simulink model "fullproject"  (R2021b)
settings: Solver=VariableStepAuto  StartTime=0.0  StopTime=0.1  RelTol=1e-3
libraries: spsMeanLib x9, spsDiodeLib x7, spsSeriesRLCBranchLib x4, spsACVoltageSourceLib x3, spsCurrentMeasurementLib x3, spsVoltageMeasurementLib x3, spsDCVoltageSourceLib x2, spsIGBTLib x1, spspowerguiLib x1
settings Model: Creator=yorga  LastModifiedBy=mluser

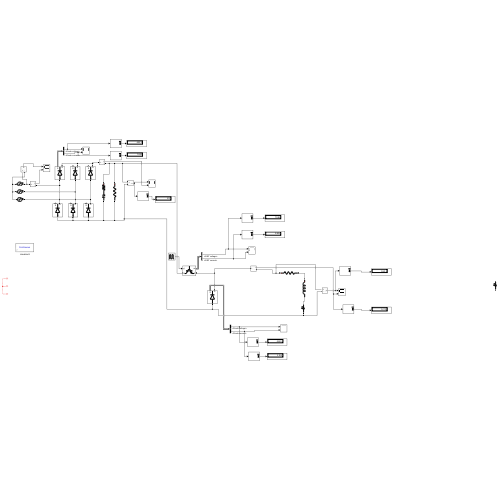
[thumbnail: Simulink's stored preview of the top-level diagram]
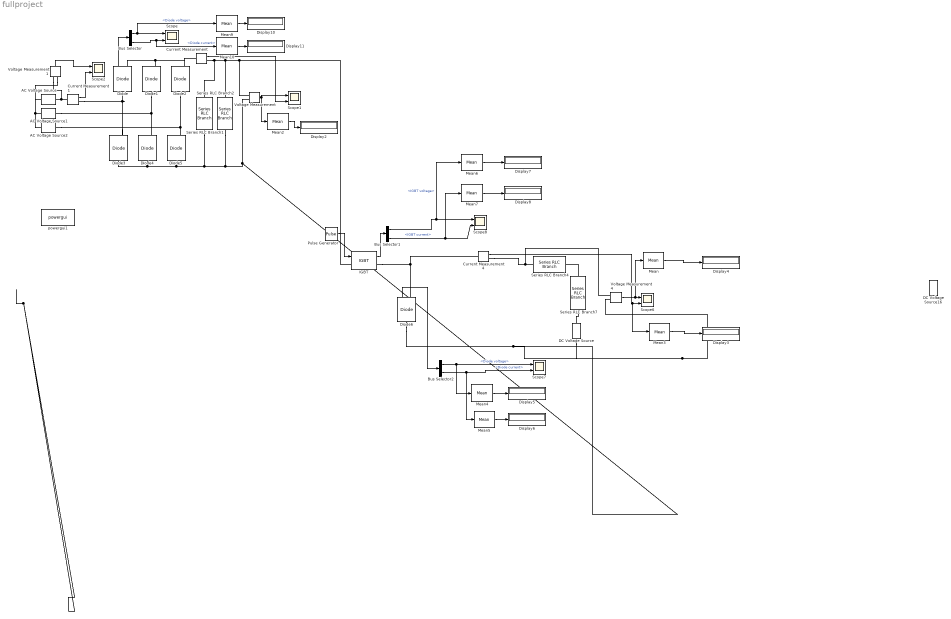
== system fullproject ==
  AC Voltage Source : spsACVoltageSourceLib/AC Voltage Source  Amplitude=100*sqrt(2)  Phase=0  Frequency=50  SampleTime=1e-4  Measurements=None  BusType=swing  Pref=10e3  Qref=0  Qmin=-inf  Qmax=+inf
  AC Voltage Source1 : spsACVoltageSourceLib/AC Voltage Source  Amplitude=100*sqrt(2)  Phase=-120  Frequency=50  SampleTime=1e-4  Measurements=None  BusType=swing  Pref=10e3  Qref=0  Qmin=-inf  Qmax=+inf
  AC Voltage Source2 : spsACVoltageSourceLib/AC Voltage Source  Amplitude=100*sqrt(2)  Phase=120  Frequency=50  SampleTime=1e-4  Measurements=None  BusType=swing  Pref=10e3  Qref=0  Qmin=-inf  Qmax=+inf
  Bus Selector : BusSelector  OutputSignals=Diode voltage,Diode current
  Bus Selector1 : BusSelector  OutputSignals=IGBT voltage,IGBT current
  Bus Selector2 : BusSelector  OutputSignals=Diode voltage,Diode current
  Current Measurement : spsCurrentMeasurementLib/Current Measurement  PhasorSimulation=off  OutputType=Complex  PSBequivalent=0
  Current Measurement1 : spsCurrentMeasurementLib/Current Measurement  PhasorSimulation=off  OutputType=Complex  PSBequivalent=0
  Current Measurement4 : spsCurrentMeasurementLib/Current Measurement  PhasorSimulation=off  OutputType=Complex  PSBequivalent=0
  DC Voltage Source : spsDCVoltageSourceLib/DC Voltage Source  Amplitude=157.08  Measurements=None
  DC Voltage Source16 : spsDCVoltageSourceLib/DC Voltage Source  Amplitude=157.08  Measurements=None
  Diode{,1..5} (6 alike) : spsDiodeLib/Diode  Ron=0  Lon=0  Vf=1.46  IC=0  UseSnubber=0  Rs=inf  Cs=0  Measurements=on
  Diode6 : spsDiodeLib/Diode  Ron=0.01  Lon=0  Vf=0  IC=0  UseSnubber=0  Rs=0  Cs=0  Measurements=on
  Display{2..8,10..11} (9 alike) : Display
  IGBT : spsIGBTLib/IGBT  Ron=0.001  Lon=0  Vf=0  Tf=1e-6  Tt=2e-6  IC=0  Rs=0  Cs=0  Measurements=on
  Mean{,2..7,9..10} (9 alike) : spsMeanLib/Mean  Freq=60  Vinit=0  Ts=0
  Pulse Generator : DiscretePulseGenerator  PulseType=Time based  Period=0.001  PulseWidth=70
  Scope{,1..2,6..8} (6 alike) : Scope  NumInputPorts=2
  Series RLC Branch1 : spsSeriesRLCBranchLib/Series RLC Branch  LConnTagsString=__new0  RConnTagsString=__new0  BranchType=RC  Resistance=0.24  Inductance=1.5e-3  SetiL0=off  InitialCurrent=0  Capacitance=470e-6  Setx0=off  InitialVoltage=0  Measurements=None
  Series RLC Branch2 : spsSeriesRLCBranchLib/Series RLC Branch  LConnTagsString=__new0  RConnTagsString=__new0  BranchType=R  Resistance=10  Inductance=24.5e-3  SetiL0=off  InitialCurrent=0  Capacitance=1e-6  Setx0=off  InitialVoltage=0  Measurements=None
  Series RLC Branch4 : spsSeriesRLCBranchLib/Series RLC Branch  LConnTagsString=__new0  RConnTagsString=__new0  BranchType=R  Resistance=0.8  Inductance=1e-3  SetiL0=off  InitialCurrent=0  Capacitance=1e-6  Setx0=off  InitialVoltage=0  Measurements=None
  Series RLC Branch7 : spsSeriesRLCBranchLib/Series RLC Branch  LConnTagsString=__new0  RConnTagsString=__new0  BranchType=L  Resistance=1  Inductance=0.0125  SetiL0=off  InitialCurrent=0  Capacitance=1e-6  Setx0=off  InitialVoltage=0  Measurements=None
  Voltage Measurement : spsVoltageMeasurementLib/Voltage Measurement  PhasorSimulation=off  OutputType=Complex  PSBequivalent=0
  Voltage Measurement1 : spsVoltageMeasurementLib/Voltage Measurement  PhasorSimulation=off  OutputType=Complex  PSBequivalent=0
  Voltage Measurement4 : spsVoltageMeasurementLib/Voltage Measurement  PhasorSimulation=off  OutputType=Complex  PSBequivalent=0
  powergui1 : spspowerguiLib/powergui  Priority=1  SimulationMode=Continuous  SampleTime=50e-6  frequency=60  Iterations=50  frequencyindice=50  Pbase=100e6  ErrMax=1e-4  UnitsV=kV  UnitsW=MW  buscounter=0  FunctionMessages=off  echomessages=off  EnableUseOfTLC=off  CurrentSourceSwitches=off  DisableSnubberDevices=off  DisableRonSwitches=off  DisableVfSwitches=off  DisplayEquations=off  AutomaticDiscreteSolvers=off  SolverType=Tustin/Backward Euler (TBE)  Interpol=off  ExternalGateDelay=off  methode=off  Ts=100  x0status=blocks  SPID=on  SwTol=0  HookPort=off  NonlinearTolerance=1e-4  nMaxIteration=100  ContinueOnMaxIteration=off  RestoreLinks=warning  ResistiveCurrentMeasurement=off  Frange=[0:2:500]  Ylog=off  Xlog=on  ShowGrid=off  save=off  variable=ZData  structure=0  ZoomFFT=off  StartTime=0.0  cycles=1  DisplayStyle=1  fundamental=60  FreqAxis=off  MaxFrequency=1000  frequencyindicesteady=1  RmsSteady=1  display=off
  wires:
  Diode/1 -> Bus Selector/1
  Bus Selector/1 -> Mean9/1, Scope/1  "<Diode voltage>"
  Bus Selector/2 -> Mean10/1, Scope/2  "<Diode current>"
  Voltage Measurement/1 -> Scope1/1, Mean2/1
  Current Measurement/1 -> Scope1/2
  Mean2/1 -> Display2/1
  Voltage Measurement1/1 -> Scope2/1
  Current Measurement1/1 -> Scope2/2
  Pulse Generator/1 -> IGBT/1
  IGBT/1 -> Bus Selector1/1
  Voltage Measurement4/1 -> Mean/1, Scope6/1
  Current Measurement4/1 -> Mean3/1, Scope6/2
  Mean3/1 -> Display3/1
  Mean/1 -> Display4/1
  Diode6/1 -> Bus Selector2/1
  Bus Selector2/1 -> Mean4/1, Scope7/1  "<Diode voltage>"
  Bus Selector2/2 -> Mean5/1, Scope7/2  "<Diode current>"
  Mean4/1 -> Display5/1
  Mean5/1 -> Display6/1
  Bus Selector1/1 -> Mean6/1, Scope8/1  "<IGBT voltage>"
  Bus Selector1/2 -> Mean7/1, Scope8/2  "<IGBT current>"
  Mean6/1 -> Display7/1
  Mean7/1 -> Display8/1
  Mean10/1 -> Display11/1
  Mean9/1 -> Display10/1
  connections:
  AC Voltage Source1/LConn1 -- Voltage Measurement1/LConn2 -- AC Voltage Source/LConn1 -- AC Voltage Source2/LConn1
  Diode3/RConn1 -- Current Measurement1/RConn1 -- Diode/LConn1
  Diode1/LConn1 -- AC Voltage Source1/RConn1 -- Diode4/RConn1
  Diode2/LConn1 -- AC Voltage Source2/RConn1 -- Diode5/RConn1
  Current Measurement/RConn1 -- Series RLC Branch1/LConn1 -- Series RLC Branch2/LConn1 -- Voltage Measurement/LConn1 -- IGBT/LConn1
  Current Measurement1/LConn1 -- Voltage Measurement1/LConn1 -- AC Voltage Source/RConn1
  Diode/RConn1 -- Current Measurement/LConn1 -- Diode2/RConn1 -- Diode1/RConn1
  ?
  IGBT/RConn1 -- Diode6/RConn1 -- Current Measurement4/LConn1
  Current Measurement4/RConn1 -- Voltage Measurement4/LConn1 -- Series RLC Branch4/LConn1
  DC Voltage Source/RConn1 -- Series RLC Branch7/RConn1
  Series RLC Branch7/LConn1 -- Series RLC Branch4/RConn1
  Voltage Measurement/LConn2 -- Diode6/LConn1 -- DC Voltage Source/LConn1 -- Voltage Measurement4/LConn2 -- Series RLC Branch2/RConn1 -- Series RLC Branch1/RConn1 -- Diode5/LConn1 -- Diode3/LConn1 -- Diode4/LConn1
